simulink model "part_3_1"  (R2021a)
settings: Solver=VariableStepAuto  StartTime=0.0  StopTime=10.0  RelTol=1e-3
settings Model: Creator=theod  LastModifiedBy=theod

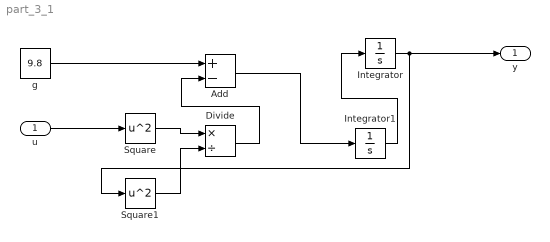
== system part_3_1 ==
  u : Inport
  Add : Sum  Inputs=+-
  Divide : Product  Inputs=*/
  Integrator : Integrator
  Integrator1 : Integrator
  Square : Math  Operator=square  SaturateOnIntegerOverflow=on
  Square1 : Math  Operator=square  SaturateOnIntegerOverflow=on
  g : Constant  Value=9.8
  y : Outport
  wires:
  Integrator1/1 -> Integrator/1
  Integrator/1 -> Square1/1, y/1
  u/1 -> Square/1
  Square/1 -> Divide/1
  Square1/1 -> Divide/2
  Divide/1 -> Add/2
  g/1 -> Add/1
  Add/1 -> Integrator1/1
